simulink library "slctrlobsolete"  (Simulink 8.9)
settings: Solver=ode45  StartTime=0.0  StopTime=10.0  RelTol=1e-3  EnableMultiTasking=on
undefined symbols (not defined in the file or in its folder): connectline
settings Model: Creator=jglass  LastModifiedBy=bxu

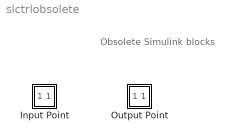
== system slctrlobsolete ==
  note: Obsolete Simulink blocks
  Input Point : Subsystem  StartFcn=connectline('start');  TreatAsAtomicUnit=on  mask(InputPoint){}
      mask help:
      | Use this block to specify the inputs of the submodel to be analyzed with the LTI Viewer for Simulink.
      |
      | You can launch the LTI Viewer by selecting "Linear Analysis" under the Tools menu.
      settings: CopyFcn=connectline('copy');  DeleteFcn=connectline('delete');  OpenFcn=connectline('open');
      mask Display: plot(33,-30,66,100,[31,38],[70,70],[34.5,34.5],[56,86],[50,50],[50,100],[50,55],[50,80],[50,45],[50,80],[50,53,55,55,55,53,50,47,44,44,44,47,50],[50,49,40,30,21,10,10,10,21,30,40,50,50],[33 44],[31 31],[56 66],[31 31])
  Output Point : Subsystem  TreatAsAtomicUnit=on  mask(OutputPoint){}
      mask help:
      | Use this block to specify the outputs of the submodel to be analyzed with the LTI Viewer for Simulink.
      |
      | You can launch the LTI Viewer by selecting "Linear Analysis" under the Tools menu.
      settings: CopyFcn=connectline('copy');  DeleteFcn=connectline('delete');  OpenFcn=connectline('open');
      mask Display: plot(33,-30,66,100,[49.5,49.5],[50,100],[50,55],[100,80],[50,45],[100,80],[46,48,51,53,53,50,48,46,46],[40,50,50,40,30,20,21,30,40],[33 44],[33 33],[53 66],[33 33])

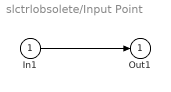
== system slctrlobsolete/Input Point ==
  In1 : Inport
  Out1 : Outport
  wires:
  In1/1 -> Out1/1

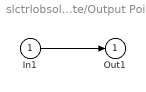
== system slctrlobsolete/Output Point ==
  In1 : Inport
  Out1 : Outport  InitialOutput=0
  wires:
  In1/1 -> Out1/1
